simulink model "DOF6_parallel"  (R2022a)
settings: Solver=VariableStepAuto  StartTime=0.0  StopTime=10.0  RelTol=1e-3
libraries: vehdynlibeom x1
settings Model: Creator=gautamd  LastModifiedBy=gautamd

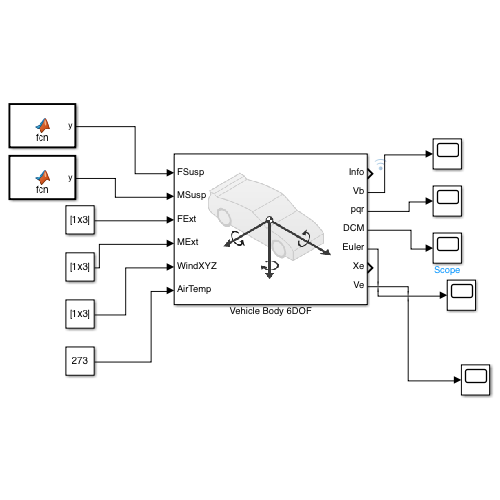
[thumbnail: Simulink's stored preview of the top-level diagram]
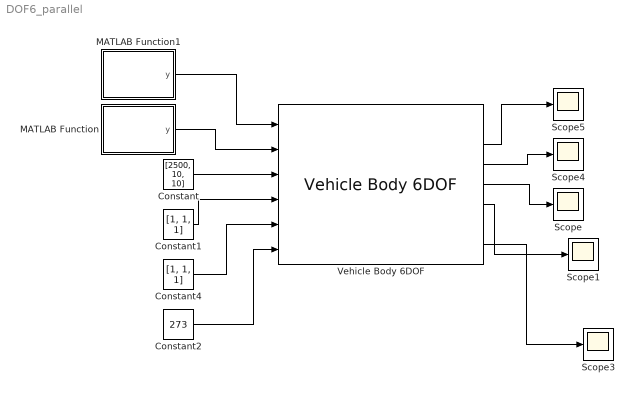
== system DOF6_parallel ==
  Constant : Constant  Value=[2500, 10, 10]  VectorParams1D=off
  Constant1 : Constant  Value=[1, 1, 1]  VectorParams1D=off
  Constant2 : Constant  Value=273
  Constant4 : Constant  Value=[1, 1, 1]  VectorParams1D=off
  MATLAB Function : MATLAB Function  TreatAsAtomicUnit=on
  MATLAB Function1 : MATLAB Function  TreatAsAtomicUnit=on
  Scope{,1,3..5} (5 alike) : Scope
  Vehicle Body 6DOF : vehdynlibeom/Vehicle Body 6DOF  extPos=on  extVel=on  extEuler=on  extRotRate=on  htchFMode=off  htchMMode=off  m=250  a=1  b=1  d=0  h=0.35  dh=1  hl=0  hh=0.1  Xe_o=[0,0,0]  xbdot_o=[0,0,0]  eul_o=[0,0,0]  p_o=[0,0,0]  Iveh=[0 0 0; 0 0 0; 0 0 0]  w=[0.9,0.9]  z1m=0  z1R=[-.25,.125,.15]  z1I=[1.4,-.2,.1;-.2,1.4,.1;.1,.1,2.25].*0  z2m=0  z2R=[1.4,0,.8]  z2I=[1.4,-.2,.1;-.2,1.4,.1;.1,.1,2.25].*0  z3m=0  z3R=[.75,-.5,.4]  z3I=[5,-.1,-2;-2,9,.1;-.1,.1,6].*0  z4m=0  z4R=[.75,.5,.4]  z4I=[5,-.1,-2;-2,9,.1;-.1,.1,6].*0  z5m=0  z5R=[1.25,-.5,.4]  z5I=[5,-.1,-2;-2,9,.1;-.1,.1,6].*0  z6m=0  z6R=[1.25,-.5,.4]  z6I=[5,-.1,-2;-2,9,.1;-.1,.1,6].*0  z7m=0  z7R=[2,0,.25]  z7I=[1.4,-.2,.1;-.2,1.4,.1;.1,.1,2.25].*0  Af=0  Cd=0  Cl=0  Cpm=0  beta_w=[0:0.001:0.001]  Cs=[0:0.001:0.001]  Cym=[0:0.001:0.001]  Pabs=101325  extTamb=on  Tair=273  g=9.81  xdot_tol=.1  longOff=0  latOff=0  vertOff=0  wrapAng=on  aMode=2
      settings: SourceProductBaseCode=VE
  wires:
  Constant/1 -> Vehicle Body 6DOF/3
  Vehicle Body 6DOF/2 -> Scope5/1
  Vehicle Body 6DOF/3 -> Scope4/1
  Vehicle Body 6DOF/7 -> Scope3/1
  Vehicle Body 6DOF/4 -> Scope/1
  Vehicle Body 6DOF/5 -> Scope1/1
  Constant1/1 -> Vehicle Body 6DOF/4
  Constant2/1 -> Vehicle Body 6DOF/6
  MATLAB Function1/1(y) -> Vehicle Body 6DOF/1
  Constant4/1 -> Vehicle Body 6DOF/5
  MATLAB Function/1(y) -> Vehicle Body 6DOF/2

== matlab function DOF6_parallel/MATLAB Function ==
  data: y output
function y = fcn()

y = [1, 2, 3, 4; 1, 2, 3, 4; 1, 2, 3, 4];

== matlab function DOF6_parallel/MATLAB Function1 ==
  data: y output
function y = fcn()

y = [1, 2, 3, 4; 1, 2, 3, 4; 1, 2, 3, 4];
